simulink model "AircraftModel"  (R2023b)
settings: Solver=VariableStepAuto  StartTime=0.0  StopTime=TF  RelTol=1e-3
values from neighbouring files (symbols this model uses):
  init = [longitude0;latitude0;altitude0;phi0;theta0;psi0;U0;V0;W0;P0;Q0;R0]    [Runaeromodel.m]
  maxAileronDeflection = 25*(pi/180)    (= 0.436332312999)    [Runaeromodel.m]
  maxElevatorDeflection = 10*(pi/180)    (= 0.174532925199)    [Runaeromodel.m]
  maxRudderDeflection = 30*(pi/180)    (= 0.523598775598)    [Runaeromodel.m]
  U_0 = [deltaT10;deltaT20;deltaA0;deltaE0;deltaR0]    [Runaeromodel.m]
undefined symbols (not defined in the file or in its folder): aeromodel, PW2040
libraries: aerolibfltsims x2, aerolibanimutils x1
settings Model: Creator=Reza  LastModifiedBy=quich
settings OptimizationCC: ReuseModelBlockBuffer=off
settings DebuggingCC: UnconnectedInputMsg=warning  UnconnectedOutputMsg=warning  UnconnectedLineMsg=warning
settings ModelReferenceCC: EnableRefExpFcnMdlSchedulingChecks=on
settings RTWCC: DLArmComputeVersion=19.05

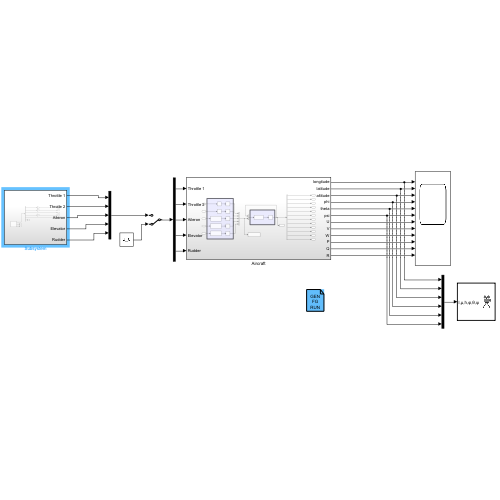
[thumbnail: Simulink's stored preview of the top-level diagram]
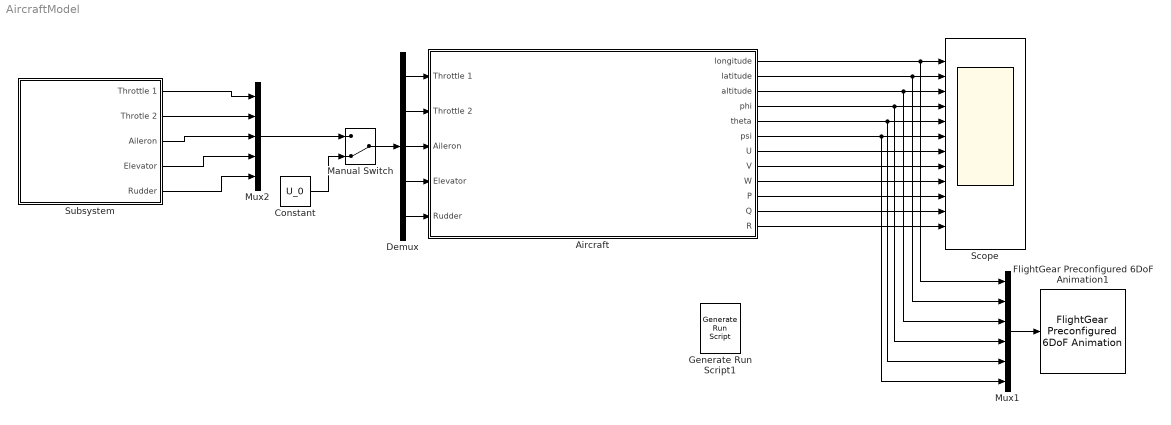
== system AircraftModel ==
  Aircraft : Subsystem
  Constant : Constant  Value=U_0
  Demux : Demux  Outputs=5
  FlightGear Preconfigured 6DoF Animation1 : aerolibfltsims/FlightGear Preconfigured 6DoF Animation  xFlightGearVersion=v2019.1  DestinationIpAddress=127.0.0.1  DestinationPort=5502  SampleTime=1/30  packetVersion=24
  Generate Run Script1 : aerolibfltsims/Generate Run Script  Architecture=Win64  dataFlow=Send  GeometryModelName=757-200-PW2040  AirportId=YYZ  RunwayId=10L  InitialAltitude=7224  InitialHeading=0  OffsetDistance=4.72  OffsetAzimuth=0  InstallScenery=on  DisableShaders=on  OriginAddress=127.0.0.1  DestinationPort=5502  OriginPort=5505  LocalAddress=127.0.0.1  OutputFileName=runfg.bat  FlightGearBaseDirectory=C:\Program Files\FlightGear 2020.3
  Manual Switch : ManualSwitch  CurrentSetting=0
  Mux1 : Mux  Inputs=6
  Mux2 : Mux  Inputs=5
  Scope : Scope  NumInputPorts=12
  Subsystem : Subsystem
  wires:
  Constant/1 -> Manual Switch/2
  Mux2/1 -> Manual Switch/1
  Manual Switch/1 -> Demux/1
  Subsystem/1(Throttle 1) -> Mux2/1
  Aircraft/7(U) -> Scope/7
  Aircraft/8(V) -> Scope/8
  Aircraft/9(W) -> Scope/9
  Aircraft/10(P) -> Scope/10
  Aircraft/11(Q) -> Scope/11
  Aircraft/12(R) -> Scope/12
  Demux/4 -> Aircraft/4(Elevator)
  Demux/1 -> Aircraft/1(Throttle 1)
  Demux/2 -> Aircraft/2(Throttle 2)
  Demux/3 -> Aircraft/3(Aileron)
  Demux/5 -> Aircraft/5(Rudder)
  Subsystem/3(Aileron) -> Mux2/3
  Subsystem/4(Elevator) -> Mux2/4
  Subsystem/5(Rudder) -> Mux2/5
  Aircraft/4(phi) -> Mux1/4, Scope/4
  Aircraft/6(psi) -> Mux1/6, Scope/6
  Aircraft/3(altitude) -> Mux1/3, Scope/3
  Aircraft/5(theta) -> Mux1/5, Scope/5
  Mux1/1 -> FlightGear Preconfigured 6DoF Animation1/1
  Aircraft/1(longitude) -> Scope/1, Mux1/1
  Aircraft/2(latitude) -> Scope/2, Mux1/2
  Subsystem/2(Throtle 2) -> Mux2/2

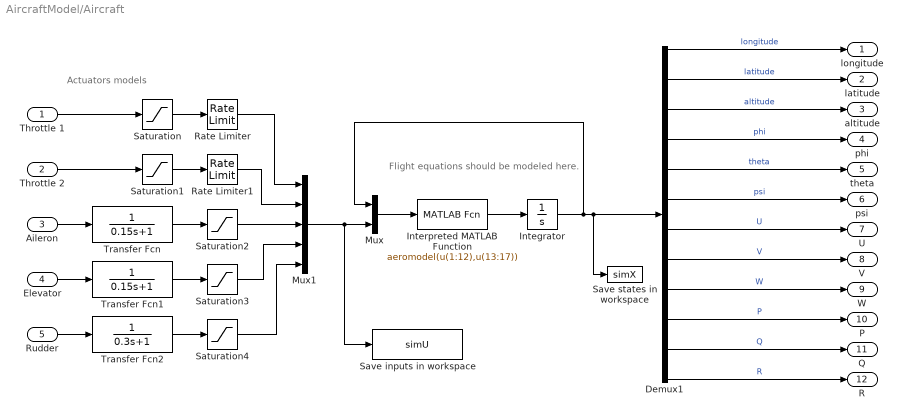
== system AircraftModel/Aircraft ==
  note: Flight equations should be
      | modeled here.
  note: Actuators models
  Throttle 1 : Inport
  Throttle 2 : Inport  Port=2
  Aileron : Inport  Port=3
  Elevator : Inport  Port=4
  Rudder : Inport  Port=5
  Demux1 : Demux  Outputs=12
  Integrator : Integrator  InitialCondition=init
  Interpreted MATLAB Function : MATLABFcn  MATLABFcn=aeromodel(u(1:12),u(13:17))
  Mux : Mux  Inputs=2
  Mux1 : Mux  Inputs=5
  Rate Limiter : RateLimiter  RisingSlewLimit=1.6  FallingSlewLimit=-1.6  SampleTimeMode=inherited
  Rate Limiter1 : RateLimiter  RisingSlewLimit=1.6  FallingSlewLimit=-1.6  SampleTimeMode=inherited
  Saturation : Saturate  UpperLimit=1*(pi/180)  LowerLimit=0.5*(pi/180)
  Saturation1 : Saturate  UpperLimit=1*(pi/180)  LowerLimit=0.5*(pi/180)
  Saturation2 : Saturate  UpperLimit=25*(pi/180)  LowerLimit=-25*(pi/180)
  Saturation3 : Saturate  UpperLimit=10*(pi/180)  LowerLimit=-25*(pi/180)
  Saturation4 : Saturate  UpperLimit=30*(pi/180)  LowerLimit=-30*(pi/180)
  Save inputs in workspace : ToWorkspace  VariableName=simU  SaveFormat=Timeseries  SampleTime=-1
  Save states in workspace : ToWorkspace  VariableName=simX  SaveFormat=Timeseries  SampleTime=-1
  Transfer Fcn : TransferFcn  Denominator=[0.15 1]
  Transfer Fcn1 : TransferFcn  Denominator=[0.15 1]
  Transfer Fcn2 : TransferFcn  Denominator=[0.3 1]
  longitude : Outport
  latitude : Outport  Port=2
  altitude : Outport  Port=3
  phi : Outport  Port=4
  theta : Outport  Port=5
  psi : Outport  Port=6
  U : Outport  Port=7
  V : Outport  Port=8
  W : Outport  Port=9
  P : Outport  Port=10
  Q : Outport  Port=11
  R : Outport  Port=12
  wires:
  Integrator/1 -> Mux/1, Save states in workspace/1, Demux1/1
  Rate Limiter/1 -> Mux1/1
  Saturation4/1 -> Mux1/5
  Rate Limiter1/1 -> Mux1/2
  Demux1/6 -> psi/1  "psi"
  Saturation/1 -> Rate Limiter/1
  Mux1/1 -> Save inputs in workspace/1, Mux/2
  Demux1/2 -> latitude/1  "latitude"
  Demux1/10 -> P/1  "P"
  Aileron/1 -> Transfer Fcn/1
  Saturation2/1 -> Mux1/3
  Saturation3/1 -> Mux1/4
  Demux1/7 -> U/1  "U"
  Throttle 2/1 -> Saturation1/1
  Saturation1/1 -> Rate Limiter1/1
  Demux1/5 -> theta/1  "theta"
  Demux1/3 -> altitude/1  "altitude"
  Demux1/1 -> longitude/1  "longitude"
  Throttle 1/1 -> Saturation/1
  Elevator/1 -> Transfer Fcn1/1
  Rudder/1 -> Transfer Fcn2/1
  Demux1/4 -> phi/1  "phi"
  Demux1/9 -> W/1  "W"
  Demux1/11 -> Q/1  "Q"
  Demux1/12 -> R/1  "R"
  Demux1/8 -> V/1  "V"
  Transfer Fcn/1 -> Saturation2/1
  Transfer Fcn1/1 -> Saturation3/1
  Transfer Fcn2/1 -> Saturation4/1
  Interpreted MATLAB Function/1 -> Integrator/1
  Mux/1 -> Interpreted MATLAB Function/1

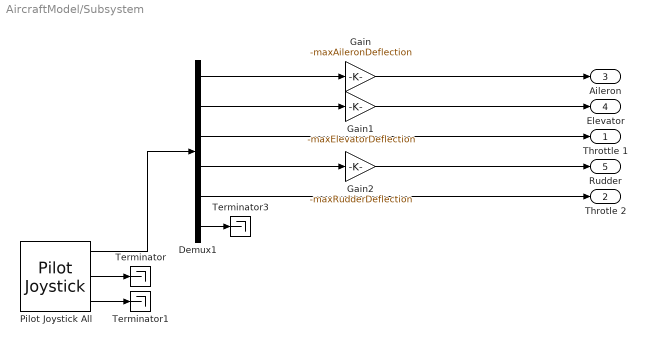
== system AircraftModel/Subsystem ==
  Demux1 : Demux  Outputs=6
  Gain : Gain  Gain=-maxAileronDeflection
  Gain1 : Gain  Gain=-maxElevatorDeflection
  Gain2 : Gain  Gain=-maxRudderDeflection
  Pilot Joystick All : aerolibanimutils/Pilot Joystick  JoystickID=Joystick1  OutputConfiguration=AllOutputs  SampleTime=1/30
  Terminator : Terminator
  Terminator1 : Terminator
  Terminator3 : Terminator
  Throttle 1 : Outport
  Throtle 2 : Outport  Port=2
  Aileron : Outport  Port=3
  Elevator : Outport  Port=4
  Rudder : Outport  Port=5
  wires:
  Demux1/3 -> Throttle 1/1
  Pilot Joystick All/3 -> Terminator1/1
  Demux1/4 -> Gain2/1
  Demux1/2 -> Gain1/1
  Pilot Joystick All/1 -> Demux1/1
  Demux1/5 -> Throtle 2/1
  Demux1/6 -> Terminator3/1
  Pilot Joystick All/2 -> Terminator/1
  Demux1/1 -> Gain/1
  Gain/1 -> Aileron/1
  Gain1/1 -> Elevator/1
  Gain2/1 -> Rudder/1
